simulink model "dc_microgrid"  (Simulink 7.3)
settings: Solver=ode45  StartTime=0.0  StopTime=1  RelTol=1e-3
InitFcn:
  | % The chosen Target in the Coder Options window must match the selected LaunchPad.
  | % Set the variable 'type_evm' to the following strings to choose a specific target:
  | 
  | % Processor selection for 1. ISOP DAB Converter:
  | 
  | type_evm_isop_1 = 'TI2806x'; % TI2806x Piccolo Launchpad
  | 
  | % Processor selection for 2. ISOP DAB Converter:
  | 
  | type_evm_isop_2 = 'TI2806x'; % TI2806x Piccolo Launchpad
  | 
  | % Processor selection for Grid Interface Converter:
  | 
  | type_evm_gic = 'TI2837xD'; % TI2837xD Delfino Launchpad
  | 
  | % Configure I/O based on processor
  | switch(type_evm_isop_1)
  | case 'TI2806x'
  | % Configuration for TI2806x
  | % Analog In\Out Configuration
  | % 3.3V AO Configuration
  | BSS1.plant.I_LV_max = 400;
  | BSS1.plant.I_LV_range = 3.3;
  | BSS1.plant.I_LV_scale = BSS1.plant.I_LV_range/2/BSS1.plant.I_LV_max;
  | BSS1.plant.I_LV_offset = 3.3/2;
  | % 3.3V AO Configuration
  | BSS1.plant.V_LV_max = 120*1.25;
  | BSS1.plant.V_LV_range = 3.3;
  | BSS1.plant.V_LV_scale = BSS1.plant.V_LV_range/BSS1.plant.V_LV_max;
  | BSS1.plant.V_LV_offset = 0;
  | % 3.3V AO Configuration
  | BSS1.plant.V_HV_max = 375*1.25;
  | BSS1.plant.V_HV_range = 3.3;
  | BSS1.plant.V_HV_scale = BSS1.plant.V_HV_range/BSS1.plant.V_HV_max;
  | BSS1.plant.V_HV_offset = 0;
  | % 3.3V AO Configuration
  | BSS1.plant.V_C_max = 375*1.25;
  | BSS1.plant.V_C_range = 3.3;
  | BSS1.plant.V_C_scale = BSS1.plant.V_C_range/2/BSS1.plant.V_C_max;
  | BSS1.plant.V_C_offset = BSS1.plant.V_C_range/2;
  | BSS1.plant.PWM_RTBox_Cap1 = [0 1 2 3];
  | BSS1.plant.PWM_RTBox_Cap2 = [16 17 18 19];
  | BSS1.plant.DI_RTBox_Eni = 29; % Global enable emulated by sliding switch
  | BSS1.plant.DO_RTBox_Eno = 4; % Global enable DO
  | BSS1.plant.DI_RTBox_Tzi = 28; % TZ1 DI emulated with sliding switch
  | BSS1.plant.DO_RTBox_Tzo = 2; % TZ1 DO
  | BSS1.plant.DI_RTBox_Power = 22; % Powerstage enable DI
  | BSS1.plant.DO_RTBox_Enabled = 29; %
  | BSS1.plant.DO_RTBox_TzLED = 28; %
  | BSS1.plant.DO_RTBox_LED = 30; %
  | BSS1.ctr.DSP_ADC_channels = [7 9 2 10 0 8 1];
  | BSS1.ctr.DSP_ADC_scale = [1/BSS1.plant.V_LV_scale 1/BSS1.plant.V_HV_scale 1/BSS1.plant.I_LV_scale 1/BSS1.plant.V_HV_scale 1/BSS1.plant.I_LV_scale 1/BSS1.plant.V_C_scale 1/BSS1.plant.V_C_scale];
  | BSS1.ctr.DSP_ADC_offset = [0 0 -BSS1.plant.I_LV_offset/BSS1.plant.I_LV_scale 0 -BSS1.plant.I_LV_offset/BSS1.plant.I_LV_scale -BSS1.plant.V_C_offset/BSS1.plant.V_C_scale -BSS1.plant.V_C_offset/BSS1.plant.V_C_scale];
  | 
  | BSS1.ctr.DO_DSP_LED = 34; % Blinking LED on LaunchPad XL
  | BSS1.ctr.DI_DSP_En = 13; % Global enable DI
  | BSS1.ctr.PWR_DSP_GPIO = 27; % Powerstage enable DO
  | BSS1.ctr.TZ_DSP_Tz1 = 12; % TZ1 DI
  | 
  | otherwise
  | error('Unknown evaluation module selection, please choose ''TI2806x''.')
  | end
  | 
  | % Configure I/O based on processor
  | switch(type_evm_isop_2)
  | case 'TI2806x'
  | % Configuration for TI2806x
  | % Analog In\Out Configuration
  | % 3.3V AO Configuration
  | BSS2.plant.I_LV_max = 400;
  | BSS2.plant.I_LV_range = 3.3;
  | BSS2.plant.I_LV_scale = BSS2.plant.I_LV_range/2/BSS2.plant.I_LV_max;
  | BSS2.plant.I_LV_offset = 3.3/2;
  | % 3.3V AO Configuration
  | BSS2.plant.V_LV_max = 120*1.25;
  | BSS2.plant.V_LV_range = 3.3;
  | BSS2.plant.V_LV_scale = BSS2.plant.V_LV_range/BSS2.plant.V_LV_max;
  | BSS2.plant.V_LV_offset = 0;
  | % 3.3V AO Configuration
  | BSS2.plant.V_HV_max = 375*1.25;
  | BSS2.plant.V_HV_range = 3.3;
  | BSS2.plant.V_HV_scale = BSS2.plant.V_HV_range/BSS2.plant.V_HV_max;
  | BSS2.plant.V_HV_offset = 0;
  | % 3.3V AO Configuration
  | BSS2.plant.V_C_max = 375*1.25;
  | BSS2.plant.V_C_range = 3.3;
  | BSS2.plant.V_C_scale = BSS2.plant.V_C_range/2/BSS2.plant.V_C_max;
  | BSS2.plant.V_C_offset = BSS2.plant.V_C_range/2;
  | BSS2.plant.PWM_RTBox_Cap1 = [0 1 2 3];
  | BSS2.plant.PWM_RTBox_Cap2 = [16 17 18 19];
  | BSS2.plant.DI_RTBox_Eni = 29; % Global enable emulated by sliding switch
  | BSS2.plant.DO_RTBox_Eno = 4; % Global enable DO
  | BSS2.plant.DI_RTBox_Tzi = 28; % TZ1 DI emulated with sliding switch
  | BSS2.plant.DO_RTBox_Tzo = 2; % TZ1 DO
  | BSS2.plant.DI_RTBox_Power = 22; % Powerstage enable DI
  | BSS2.plant.DO_RTBox_Enabled = 29; %
  | BSS2.plant.DO_RTBox_TzLED = 28;
  | BSS2.plant.DO_RTBox_LED = 30;
  | BSS2.ctr.DSP_ADC_channels = [7 9 2 10 0 8 1];
  | BSS2.ctr.DSP_ADC_scale = [1/BSS2.plant.V_LV_scale 1/BSS2.plant.V_HV_scale 1/BSS2.plant.I_LV_scale 1/BSS2.plant.V_HV_scale 1/BSS2.plant.I_LV_scale 1/BSS2.plant.V_C_scale 1/BSS2.plant.V_C_scale];
  | BSS2.ctr.DSP_ADC_offset = [0 0 -BSS2.plant.I_LV_offset/BSS2.plant.I_LV_scale 0 -BSS2.plant.I_LV_offset/BSS2.plant.I_LV_scale -BSS2.plant.V_C_offset/BSS2.plant.V_C_scale -BSS2.plant.V_C_offset/BSS2.plant.V_C_scale];
  | 
  | BSS2.ctr.DO_DSP_LED = 34; % Blinking LED on LaunchPad XL
  | BSS2.ctr.DI_DSP_En = 13; % Global enable DI
  | BSS2.ctr.PWR_DSP_GPIO = 27; % Powerstage enable DO
  | BSS2.ctr.TZ_DSP_Tz1 = 12; % TZ1 DI
  | otherwise
  | error('Unknown evaluation module selection, please choose ''TI2806x''.')
  | end
  | 
  | 
  | 
  | % Configure I/O based on processor
  | switch(type_evm_gic)
  | case 'TI2837xD'
  | % Configuration for TI2837xD
  | GIC.plant.AO_RTBox_Ig = [6 5 4];
  | GIC.plant.AO_RTBox_Vdc = 13;
  | GIC.plant.AO_RTBox_Vmid = 12;
  | GIC.plant.AO_RTBox_Vg = [3 2 1];
  | 
  | GIC.plant.DI_RTBox_Power = 29;
  | GIC.plant.DI_RTBox_Br = 30;
  | GIC.plant.DI_RTBox_FRT = 27;
  | 
  | GIC.plant.DO_RTBox_Power = 4;
  | GIC.plant.DO_RTBox_LED = 31;
  | GIC.plant.DO_RTBox_Enabled = 29;
  | GIC.plant.PWM_RTBox_CapA = [0 3 1 2];
  | GIC.plant.PWM_RTBox_CapB = [4 17 5 16];
  | GIC.plant.PWM_RTBox_CapC = [18 21 19 20];
  | % Analog In/Out Configuration
  | GIC.plant.ADCfull = 3.3;
  | % DC voltage sensing
  | GIC.plant.Vdc.max = 1000;
  | GIC.plant.Vdc.K = GIC.plant.ADCfull / GIC.plant.Vdc.max;
  | % DC current sensing
  | GIC.plant.Idc.max = 200;
  | GIC.plant.Idc.K = GIC.plant.ADCfull / GIC.plant.Idc.max;
  | GIC.plant.Idc.O = GIC.plant.ADCfull / 2.0;
  | % AC current
  | GIC.plant.Iph.max = 400;
  | GIC.plant.Iph.K = GIC.plant.ADCfull / GIC.plant.Iph.max ;
  | GIC.plant.Iph.O = GIC.plant.ADCfull / 2.0;
  | % AC voltage
  | GIC.plant.Vph.max = 1000;
  | GIC.plant.Vph.K = GIC.plant.ADCfull / GIC.plant.Vph.max;
  | GIC.plant.Vph.O = GIC.plant.ADCfull / 2.0;
  | % ADC channels
  | GIC.ctr.ADCA = [3 2];
  | GIC.ctr.ADCB = [3 2 4];
  | GIC.ctr.ADCC = [3 2 4];
  | % ADC scale and offset
  | GIC.ctr.ADCC_scale = [1/GIC.plant.Vph.K 1/GIC.plant.Iph.K 1/GIC.plant.Vdc.K];
  | GIC.ctr.ADCC_offset = [-GIC.plant.Vph.O/GIC.plant.Vph.K -GIC.plant.Iph.O/GIC.plant.Iph.K 0];
  | GIC.ctr.ADCB_scale = [1/GIC.plant.Vph.K 1/GIC.plant.Iph.K 1/GIC.plant.Vdc.K];
  | GIC.ctr.ADCB_offset = [-GIC.plant.Vph.O/GIC.plant.Vph.K -GIC.plant.Iph.O/GIC.plant.Iph.K 0] ;
  | GIC.ctr.ADCA_scale = [1/GIC.plant.Vph.K 1/GIC.plant.Iph.K];
  | GIC.ctr.ADCA_offset = [-GIC.plant.Vph.O/GIC.plant.Vph.K -GIC.plant.Iph.O/GIC.plant.Iph.K];
  | %
  | GIC.ctr.PWR_DSP_GPIO = 16;
  | %
  | GIC.ctr.PWM_DSP_PWM = [1:6];
  | %
  | GIC.ctr.DI_DSP_En = 24;
  | GIC.ctr.DO_DSP_FRT = 58;
  | 
  | otherwise
  | error('Unknown evaluation module selection, please choose ''TI2837xD''.')
  | end
  | 
  | DCgrid.plant.time_scaling = 1; % Time scaling for PV production, CPL and Grid fault
  | 
  | % PV Data for realistic scenario
  | DCgrid.plant.pv_data_vector = [0.00000 0.00000 0.00000 0.00000 0.00000 0.00000 0.00000 0.00000 0.00000 0.00000 0.00000 0.00000 0.00000 0.00000 0.00000 0.00000 0.00000 0.00000 0.00000 0.00000 0.00000 0.00000 0.00000 0.00000 0.00000 0.00000 0.00000 0.00000 0.00000 0.00000 0.00000 0.00000 0.00000 0.00000 0.00000 0.00000 0.00000 0.00000 0.00000 0.00000 0.00000 0.00000 0.00000 0.00000 0.00000 0.00000 0.00000 0.00000 0.00000 0.00000 0.00000 ...
  | 0.00000 0.00000 0.00000 0.00000 0.00000 0.00000 0.00000 0.00118 0.00069 0.00148 0.00042 0.00217 0.00235 0.00917 0.04586 0.08611 0.13475 0.19584 0.21060 0.22702 0.24555 0.30298 0.34206 0.41668 0.47215 0.54021 0.57121 0.61637 0.65545 0.68474 0.74728 0.75041 0.79355 0.00002 0.00002 0.87414 0.86653 0.87950 0.85384 0.84579 1.02102 0.82404 0.92416 0.93231 0.92406 0.93681 0.92926 0.92012 0.92773 0.91514 0.87933 ...
  | 0.93935 1.03093 1.04328 0.63428 0.53304 0.65434 0.66678 0.98482 0.45313 0.30253 0.36111 0.32828 0.34596 0.48013 0.41025 0.26031 0.24632 0.14307 0.10560 0.11837 0.19274 0.14353 0.13194 0.11903 0.04647 0.06786 0.13197 0.13824 0.09205 0.01515 0.00108 0.04813 0.04061 0.00028 0.00124 0.00216 0.00144 0.00220 0.00108 0.00051 0.00142 0.00149 0.00250 0.00775 0.04074 0.06619 0.05964 0.09909 0.09498 0.11656 0.13997 ...
  | 0.34046 0.27423 0.46071 0.43367 0.44145 0.29370 0.35223 0.35924 0.37953 0.57478 1.23262 0.67266 0.37461 0.50523 0.51200 1.31944 0.29329 0.58777 0.57749 0.58444 0.52717 0.25440 0.26710 0.41560 0.42609 0.28574 0.30071 0.39256 0.21140 0.15896 0.20298 0.18366 0.13576 0.17928 0.17817 0.30268 0.12528 0.07170 0.03283 0.03101 0.01341 0.01239 0.00078 0.00078 0.00120 0.00104 0.00290 0.01139 0.02320 0.06571 0.08867 ...
  | 0.15329 0.20732 0.21715 0.29141 0.35767 0.44814 0.53036 0.57656 0.66894 0.70469 0.77576 0.81051 0.83082 0.86134 0.89329 0.92838 0.94508 0.95669 0.97510 0.98210 0.98644 1.00879 0.99010 0.98902 0.99907 0.98015 0.96248 0.95868 0.94567 0.93586 0.92815 0.88212 0.87967 0.83723 0.82389 0.79127 0.76338 0.72543 0.69345 0.00000 0.00000 0.60718 0.55620 0.50278 0.45602 0.37596 0.32055 0.28157 0.23485 0.18765 0.14784 0.09659 ...
  | 0.05671 0.01581 0.00881 0.00718 0.00385 0.00398 0.00104 0.00159 0.00096 0.00130 0.00053 0.00093 0.00261 0.02322 0.05124 0.11010 0.17379 0.20935 0.25035 0.32525 0.41563 0.51662 0.56969 0.66024 0.71703 0.75227 0.79300 0.83388 0.86196 0.87870 0.91693 0.91632 0.92747 0.93203 0.94496 0.95264 0.96134 0.96371 0.96165 0.95235 0.94653 0.94026 0.91655 0.90636 0.88432 0.86209 0.83357 0.80859 0.77703 0.75426 0.71557 0.68176 ...
  | 0.64311 0.59763 0.55148 0.51006 0.46500 0.41605 0.36002 0.30248 0.25560 0.20023 0.15469 0.10653 0.05998 0.03369 0.00468 0.00333 0.00368 0.00195 0.00121 0.00048 0.00062 0.00133];
  | DCgrid.plant.time_vector = [0.00000 0.00308 0.00615 0.00923 0.01231 0.01538 0.01846 0.02154 0.02462 0.02769 0.03077 0.03385 0.03692 0.04000 0.04308 0.04615 0.04923 0.05231 0.05538 0.05846 0.06154 0.06462 0.06769 0.07077 0.07385 0.07385 0.07692 0.08000 0.08308 0.08615 0.08923 0.09231 0.09538 0.09846 0.10154 0.10462 0.10769 0.11077 0.11385 0.11692 0.12000 0.12308 0.12308 0.12615 0.12923 0.13231 0.13538 0.13846 0.14154 0.14462 0.14769 ...
  | 0.15077 0.15385 0.15692 0.16000 0.16308 0.16615 0.16923 0.17231 0.17538 0.17846 0.18154 0.18462 0.18769 0.19077 0.19385 0.19692 0.20000 0.20308 0.20615 0.20923 0.21231 0.21538 0.21846 0.22154 0.22462 0.22769 0.23077 0.23385 0.23692 0.24000 0.24308 0.24615 0.24923 0.25231 0.25538 0.25538 0.25846 0.26154 0.26462 0.26769 0.27077 0.27385 0.27692 0.28000 0.28308 0.28615 0.28923 0.29231 0.29538 0.29846 0.30154 ...
  | 0.30462 0.30769 0.31077 0.31385 0.31692 0.32000 0.32308 0.32615 0.32923 0.33231 0.33538 0.33846 0.34154 0.34462 0.34769 0.35077 0.35385 0.35692 0.36000 0.36308 0.36615 0.36923 0.37231 0.37538 0.37846 0.38154 0.38462 0.38769 0.39077 0.39385 0.39692 0.40000 0.40308 0.40615 0.40923 0.41231 0.41538 0.41846 0.42154 0.42462 0.42769 0.43077 0.43385 0.43692 0.44000 0.44308 0.44615 0.44923 0.45231 0.45538 0.45846 0.46154 ...
  | 0.46462 0.46769 0.47077 0.47385 0.47692 0.48000 0.48308 0.48615 0.48923 0.49231 0.49538 0.49846 0.50154 0.50462 0.50769 0.51077 0.51385 0.51692 0.52000 0.52308 0.52615 0.52923 0.53231 0.53538 0.53846 0.54154 0.54462 0.54769 0.55077 0.55385 0.55692 0.56000 0.56308 0.56615 0.56923 0.57231 0.57538 0.57846 0.58154 0.58462 0.58769 0.59077 0.59385 0.59692 0.60000 0.60308 0.60615 0.60923 0.61231 0.61538 0.61846 0.62154 ...
  | 0.62462 0.62769 0.63077 0.63385 0.63692 0.64000 0.64308 0.64615 0.64923 0.65231 0.65538 0.65846 0.66154 0.66462 0.66769 0.67077 0.67385 0.67692 0.68000 0.68308 0.68615 0.68923 0.69231 0.69538 0.69846 0.70154 0.70462 0.70769 0.71077 0.71385 0.71692 0.72000 0.72308 0.72615 0.72923 0.73231 0.73538 0.73846 0.74154 0.74462 0.74462 0.74769 0.75077 0.75385 0.75692 0.76000 0.76308 0.76615 0.76923 0.77231 0.77538 0.77846 ...
  | 0.78154 0.78462 0.78769 0.79077 0.79385 0.79692 0.80000 0.80308 0.80615 0.80923 0.81231 0.81538 0.81846 0.82154 0.82462 0.82769 0.83077 0.83385 0.83692 0.84000 0.84308 0.84615 0.84923 0.85231 0.85538 0.85846 0.86154 0.86462 0.86769 0.87077 0.87385 0.87692 0.88000 0.88308 0.88615 0.88923 0.89231 0.89538 0.89846 0.90154 0.90462 0.90769 0.91077 0.91385 0.91692 0.92000 0.92308 0.92615 0.92923 0.93231 0.93538 ...
  | 0.93846 0.94154 0.94462 0.94769 0.95077 0.95385 0.95692 0.96000 0.96308 0.96615 0.96923 0.97231 0.97538 0.97846 0.98154 0.98462 0.98769 0.99077 0.99385 0.99692 1.00000];
  | 
  | DCgrid.plant.PVpeak_power = 10e3; % Peak PV power used for scenario
  | 
  | DCgrid.plant.load_vector = [0.0 0.0 0.0 0.0 0.0 0.0 0.0 0.0 0.0 0.0 0.0 0.0 0.0 0.0 0.0 0.0 0.0 0.0 0.0 0.0 0.0 0.0 0.0 0.0 0.0 0.0 0.0 0.0 0.0 0.0 0.0 0.0 0.0 0.0 0.0 0.0 0.0 0.0 0.0 0.0 0.0 0.0 0.0 0.0 0.0 0.0 0.0 0.0 0.0 0.0 0.0 0.0 0.0 0.0 0.0 0.0 0.0 0.0 0.0 0.0 0.0 0.0 0.0 0.0 0.0 0.0 0.0 0.0 0.0 0.0 0.0 0.0 0.0 0.0 0.0 0.0 0.0 0.0 0.0 0.0 0.0 0.0 0.0 0.0 0.0 0.0 0.0 0.0 0.0 0.0 0.0 0.0 0.0 0.0 0.0 0.0 0.0 0.0 0.0 0.0 0.0 0.0 ...
  | 0.0 0.0 0.0 0.0 0.93 0.91 0.92 0.91 0.81 0.76 0.83 0.81 0.81 0.82 0.82 0.82 0.8 0.77 0.75 0.73 0.72 0.74 0.74 0.74 0.71 0.68 0.63 0.61 0.6 0.59 0.57 0.54 0.5 0.49 0.48 0.45 0.43 0.43 0.42 0.4 0.4 0.4 0.39 0.39 0.39 0.4 0.4 0.39 0.39 0.39 0.39 0.39 0.4 0.4 0.39 0.39 0.42 0.44 0.45 0.48 0.52 0.54 0.58 0.56 0.58 0.59 0.59 0.59 0.59 0.58 0.59 0.59 0.58 0.61 0.6 0.57 0.63 0.62 0.64 0.62 0.62 0.64 0.7 0.71 ...
  | 0.62 0.68 0.63 0.67 0.68 0.63 0.68 0.62 0.69 0.62 0.64 0.57 0.57 0.61 0.55 0.6 0.53 0.58 0.57 0.53 0.57 0.53 0.53 0.58 0.52 0.54 0.56 0.48 0.53 0.51 0.48 0.53 0.44 0.49 0.46 0.46 0.47 0.43 0.49 0.42 0.44 0.39 0.42 0.4 0.41 0.41 0.37 0.42 0.34 0.4 0.35 0.39 0.35 0.37 0.37 0.35 0.39 0.34 0.4 0.33 0.39 0.35 0.38 0.37 0.35 0.39 0.34 0.41 0.34 0.42 0.36 0.44 0.39 0.46 0.4 0.44 0.41 0.43 0.43 0.41 0.47 0.43 ...
  | 0.42 0.42 0.42 0.43 0.42 0.41 0.39 0.41 0.44 0.39 0.46 0.4 0.45 0.4 0.47 0.48 0.45 0.49 0.43 0.52 0.5 0.5 0.49 0.49 0.5 0.5 0.45 0.49 0.45 0.52 0.45 0.48 0.5 0.44 0.5 0.45 0.46 0.5 0.45 0.5 0.47 0.46 0.52 0.45 0.49 0.47 0.44 0.51 0.45 0.49 0.48 0.44 0.51 0.45 0.48 0.44 0.42 0.46 0.43 0.44 0.45 0.41];
  | 
  | DCgrid.plant.CPL_load = 12e3; % Constant power load in (W)
  | 
  | %% DC Power Grid
  | % General Parameters
  | DCgrid.plant.Tdisc = 5e-6; % Discretization step size of the DC grid model running on the RT Box
  | 
  | %% Battery Storage System 1 (BSS1)
  | 
  | % General Parameters
  | BSS1.plant.Tdisc = 3.5e-6; % Discretization step size for DAB plant (s)
  | BSS1.ctr.fsw = 15e3; % Switching frequency (Hz)
  | BSS1.ctr.Tdisc = 1/BSS1.ctr.fsw; % Discretization step size for Controller execution
  | 
  | % DAB Inductor Design
  | BSS1.plant.V_LV = 120; % Battery-side voltage (V)
  | BSS1.plant.V_HV = 375; % DC Grid-side voltage (V)
  | BSS1.plant.n = BSS1.plant.V_HV/BSS1.plant.V_LV; % Transformer turns ratio (p.u.)
  | BSS1.plant.Pnom = 10e3; % Nominal DAB power (W)
  | BSS1.plant.Clv = 1e-3; % Low-voltage side capacitance (F)
  | BSS1.plant.Chv = 1e-3;
  | BSS1.plant.Llv = 2e-5; % Low-voltage side inductor (H)
  | BSS1.plant.Rllv = 0.1; % Winding resistance of low-voltage side inductor (Ohm)
  | BSS1.plant.Rtot = 0.1; % Transformer winding resistance (Ohm)
  | BSS1.plant.Ltot = BSS1.plant.n*BSS1.plant.V_HV*BSS1.plant.V_LV/(8*BSS1.ctr.fsw*BSS1.plant.Pnom); % Total longitudal inductor (H)
  | 
  | % Droop Controller
  | BSS1.ctr.Inom = BSS1.plant.Pnom/BSS1.plant.V_LV;
  | BSS1.ctr.DroopGain = 10*BSS1.plant.n;
  | 
  | % DAB Voltage Controller
  | BSS1.ctr.KpC = 2.0;
  | BSS1.ctr.SatIUp = BSS1.plant.Pnom/BSS1.plant.V_LV;
  | BSS1.ctr.SatILow = -BSS1.plant.Pnom/BSS1.plant.V_LV;
  | 
  | % DAB Current controller
  | BSS1.ctr.KpL = 0.15;
  | BSS1.ctr.KiL = 150;
  | 
  | %% Battery Storage System 2 (BSS2)
  | 
  | % General Parameters
  | BSS2.plant.Tdisc = 3.5e-6; % Discretization step size for DAB plant (s)
  | BSS2.ctr.fsw = 15e3; % Switching frequency (Hz)
  | BSS2.ctr.Tdisc = 1/BSS2.ctr.fsw; % Discretization step size for Controller execution
  | 
  | % DAB Inductor Design
  | BSS2.plant.V_LV = 120; % Battery-side voltage (V)
  | BSS2.plant.V_HV = 375; % DC Grid-side voltage (V)
  | BSS2.plant.n = BSS2.plant.V_HV/BSS2.plant.V_LV; % Transformer turns ratio (p.u.)
  | BSS2.plant.Pnom = 10e3; % Nominal DAB power (W)
  | BSS2.plant.Clv = 1e-3; % Low-voltage side capacitance (F)
  | BSS2.plant.Chv = 1e-3;
  | BSS2.plant.Llv = 2e-5; % Low-voltage side inductor (H)
  | BSS2.plant.Rllv = 0.1; % Winding resistance of low-voltage side inductor (Ohm)
  | BSS2.plant.Rtot = 0.1; % Transformer winding resistance (Ohm)
  | BSS2.plant.Ltot = BSS2.plant.n*BSS2.plant.V_HV*BSS2.plant.V_LV/(8*BSS2.ctr.fsw*BSS2.plant.Pnom); % Total longitudal inductor (H)
  | 
  | % Droop Controller
  | BSS2.ctr.Inom = BSS2.plant.Pnom/BSS2.plant.V_LV;
  | BSS2.ctr.DroopGain = BSS1.ctr.DroopGain;
  | 
  | % DAB Voltage Controller
  | BSS2.ctr.KpC = 1.0;
  | BSS2.ctr.SatIUp = BSS2.plant.Pnom/BSS2.plant.V_LV;
  | BSS2.ctr.SatILow = -BSS2.plant.Pnom/BSS2.plant.V_LV;
  | 
  | % DAB Current controller
  | BSS2.ctr.KpL = 0.5;
  | BSS2.ctr.KiL = 200;
  | 
  | %% Grid Interface Converter(GIC)
  | 
  | % General Parameters
  | GIC.ctr.fsw = 20e3; % switching frequency
  | GIC.ctr.Tdisc = 1/GIC.ctr.fsw;
  | Vgrid_rms = 230;
  | Vnom = Vgrid_rms * sqrt(2);
  | Vll = sqrt(3)*Vgrid_rms;
  | Fgrid = 50;
  | Pn = 20e3; % nominal output power 20 kW
  | Id_ref = Pn/3/Vgrid_rms*sqrt(2);
  | 
  | % Plant settings
  | 
  | GIC.plant.Tdisc = 5.0e-6; % Discretization step size of plant running on the RT Box
  | 
  | % Outputfilter parameters
  | 
  | GIC.plant.Lf = 3e-3; % filter inductance value
  | GIC.plant.Rf = 0.1; % copper resistance
  | 
  | % Current control
  | GIC.ctr.KpI = GIC.plant.Lf*GIC.ctr.fsw/3; % Kp choosen for optimally damped system
  | Ti = GIC.plant.Lf/GIC.plant.Rf; % Compensate plant time constant
  | GIC.ctr.KiI = GIC.ctr.KpI/Ti; % Compensate plant time constant
  | 
  | % Power control
  | GIC.ctr.KpP = 1/(2*Vgrid_rms*sqrt(2));
  | GIC.ctr.KiP = 1;
  | 
  | % Harmonic Compensator
  | GIC.ctr.ki6p = 150;
  | GIC.ctr.ki6m = 150;
undefined symbols (not defined in the file): plecs
settings Model: Creator=kris  LastModifiedBy=manaswini  ExtModeTrigMode=oneshot  ExtModeArmWhenConnect=off  ExtModeAutoUpdateStatusClock=off
settings DataIOCC: LimitDataPoints=off  ReturnWorkspaceOutputs=off  SignalLoggingName=sigsOut
settings OptimizationCC: BooleanDataType=off  ExpressionDepthLimit=128  InitFltsAndDblsToZero=on
settings DebuggingCC: SaveWithParameterizedLinksMsg=none  SignalResolutionControl=TryResolveAllWithWarning  SolverPrmCheckMsg=none  MultiTaskDSMMsg=warning  MultiTaskCondExecSysMsg=none  FcnCallInpInsideContextMsg=Enable All  StrictBusMsg=ErrorLevel1
settings HardwareCC: TargetHWDeviceType=32-bit Generic  TargetUnknown=on  ProdEqTarget=off
settings CodeAppCC: CustomSymbolStrType=$N$R$M_T
settings GRTTargetCC: TargetFcnLib=ansi_tfl_tmw.mat  TargetFunctionLibrary=C89/C90 (ANSI)  ModelReferenceCompliant=off

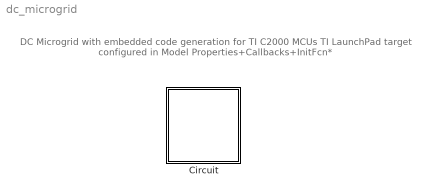
== system dc_microgrid ==
  note: DC Microgrid
      | with embedded code generation for TI C2000 MCUs
      | TI LaunchPad target configured in Model Properties+Callbacks+InitFcn*
  Circuit : Subsystem  LoadFcn=plecs('sl', 200);  InitFcn=plecs('sl', 214);  StartFcn=plecs('sl', 208);  StopFcn=plecs('sl', 209);  ClipboardFcn=plecs('sl', 212, 24);  mask(PlecsCircuit){PLECSData=<binary blob, 114692 chars, not shown>}
      mask prompts: PLECSData "PLECS Data (Do not delete or modify!)"
      mask help: Drag this block into a Simulink model to create a new electrical circuit.
      mask init:
      | % PLACE CUSTOM INITIALIZATIONS ABOVE
      | % DO NOT REMOVE
      | plecs('sl', 215);
      | % DO NOT REMOVE
      settings: CopyFcn=plecs('sl', 203);  DeleteFcn=plecs('sl', 205);  UndoDeleteFcn=plecs('sl', 206);  PreSaveFcn=plecs('sl', 211);  PostSaveFcn=plecs('sl', 201);  NameChangeFcn=plecs('sl', 210);  DestroyFcn=plecs('sl', 207);  PreCopyFcn=plecs('sl', 216);  OpenFcn=plecs('sl', 202);  ErrorFcn=plerrorfcn
      mask Display: disp('PLECS\nCircuit')

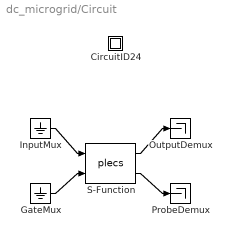
== system dc_microgrid/Circuit ==
  " CircuitID24 " : Subsystem
  " GateMux " : Ground
  " InputMux " : Ground
  " OutputDemux " : Terminator
  " ProbeDemux " : Terminator
  " S-Function " : S-Function  FunctionName=plecs  EnableBusSupport=off
  wires:
  " InputMux "/1 -> " S-Function "/1
  " GateMux "/1 -> " S-Function "/2
  " S-Function "/1 -> " OutputDemux "/1
  " S-Function "/2 -> " ProbeDemux "/1

== system dc_microgrid/Circuit/ CircuitID24  ==
